simulink model "LTO"  (R2016b)
settings: Solver=VariableStepAuto  StartTime=0.0  StopTime=t24(end)  FixedStep=0.1  RelTol=1e-3
values from neighbouring files (symbols this model uses):
  Cpmap = [CpMapDis; CpMap]    [ltoMap.m]
  I0 = 0.0    (= 0)    [Main.m]
  Ich = 5    [Main.m]
  Idis = -15    [Main.m]
  Kch = 1.0    (= 1)    [Main.m]
  Kci = 1/(D2i^2*D3i)*(Tsig0*Lc)/(Tei^2)-Rtot    [Main.m]
  KI_cmp = KR_cmp/TI_cmp    [Main.m]
  KR_cmp = (1/Rb)*(Tsigc/D2c/Tec - 1)    [Main.m]
  Lc = 0.7e-3    (= 0.0007)    [Main.m]
  P0 = 1e-1*eye(2,2)    [Main.m]
  QChg = 33.0873    [Main.m]
  Qk = [qk11 0; 0 qk22]    [Main.m]
  Qmax24Chg = 32.9569    [Main.m]
  Rc = 0.05    [Main.m]
  rk = 1e1    (= 10)    [Main.m]
  Rpmap = [RpMapDis; RpMap]    [ltoMap.m]
  T = 0.01    [Main.m]
  Tacq = 1    [Main.m]
  Tch = 1e-3    (= 0.001)    [Main.m]
  Tci = (D3i*D2i^2*Tei^3*Kci)/(Tsig0*Lc)    [Main.m]
  Tfilt = 4e-3    (= 0.004)    [Main.m]
  uc0 = 0.0    (= 0)    [Main.m]
  Udc0 = 4    [Main.m]
undefined symbols (not defined in the file or in its folder): DiscIntNeverNeededParam, dUocdT_map, T_map, xi_map
libraries: dspmtrx3 x1, simulink x1, fuzblock x1
settings Model: Creator=user  LastModifiedBy=user

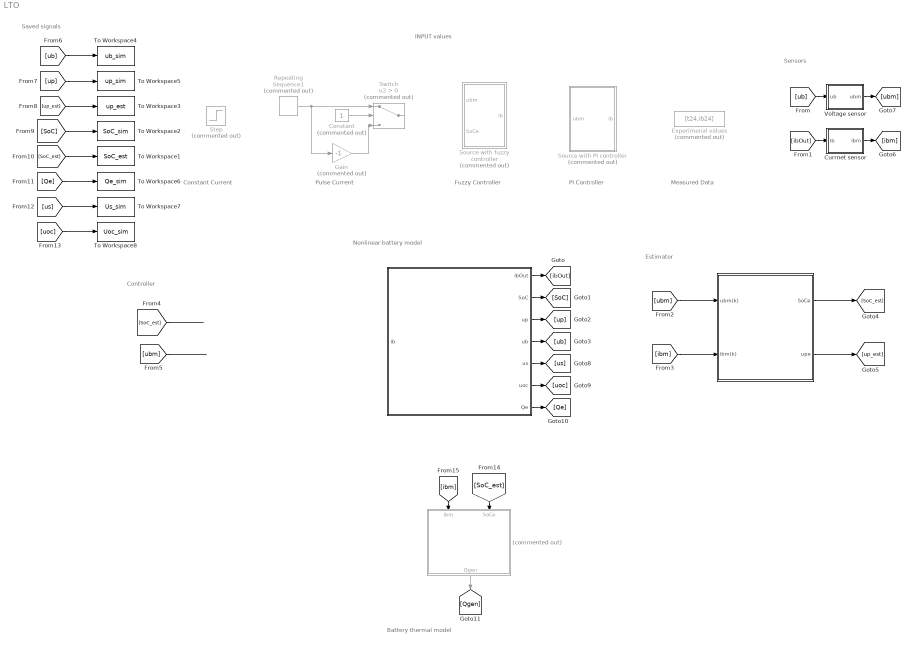
== system LTO ==
  note: Nonlinear battery model
  note: Constant Current
  note: Pulse Current
  note: Fuzzy Controller
  note: PI Controller
  note: Sensors
  note: Saved signals
  note: Measured Data
  note: INPUT values
  note: Estimator
  note: Battery thermal model
  note: Controller
  " " : Subsystem
  "  " : Subsystem  Commented=on
  "   " : Subsystem
  Constant : Constant  Commented=on
  Currnet sensor : Subsystem
  Experimenal values : FromWorkspace  Commented=on  VariableName=[t24,ib24]  SampleTime=Tacq
  Gain : Gain  Commented=on  Gain=-1
  Repeating Sequence1 : simulink/Sources/Repeating Sequence  Commented=on  rep_seq_t=[0 225 (225+2^(-40)) 300]  rep_seq_y=[Idis Idis Ich Ich]
  "Source with fuzzy controller " : Subsystem  Commented=on
  "Source with PI controller " : Subsystem  Commented=on
  Step : Step  Commented=on  After=30  SampleTime=0
  Switch : Switch  Commented=on  Criteria=u2 > Threshold
  To Workspace1 : ToWorkspace  VariableName=SoC_est  SampleTime=Tacq
  To Workspace2 : ToWorkspace  VariableName=SoC_sim  SampleTime=Tacq
  To Workspace3 : ToWorkspace  VariableName=up_est  SampleTime=Tacq
  To Workspace4 : ToWorkspace  VariableName=ub_sim  SampleTime=Tacq
  To Workspace5 : ToWorkspace  VariableName=up_sim  SampleTime=Tacq
  To Workspace6 : ToWorkspace  VariableName=Qe_sim  SampleTime=Tacq
  To Workspace7 : ToWorkspace  VariableName=Us_sim  SampleTime=Tacq
  To Workspace8 : ToWorkspace  VariableName=Uoc_sim  SampleTime=Tacq
  Voltage sensor : Subsystem
  wires:
  Constant/1 -> Switch/2
  Repeating Sequence1/1 -> Gain/1, Switch/1
  Gain/1 -> Switch/3
  " "/2(SoC) -> [SoC]
  " "/3(up) -> [up]
  " "/1("ibOut ") -> [ibOut]
  " "/4(ub) -> [ub]
  "   "/1(SoCe) -> [SoC_est]
  "   "/2(upe) -> [up_est]
  [ub] -> Voltage sensor/1(ub)
  [ibOut] -> Currnet sensor/1(ib)
  Voltage sensor/1("ubm ") -> [ubm]
  Currnet sensor/1("ibm ") -> [ibm]
  [ubm] -> "   "/1(ubm(k))
  [ibm] -> "   "/2(ibm(k))
  [ub] -> To Workspace4/1
  [up] -> To Workspace5/1
  [SoC_est] -> To Workspace1/1
  [up_est] -> To Workspace3/1
  [SoC] -> To Workspace2/1
  " "/5(us) -> [us]
  " "/6(uoc) -> [uoc]
  " "/7(Qe) -> [Qe]
  [Qe] -> To Workspace6/1
  [us] -> To Workspace7/1
  [uoc] -> To Workspace8/1
  [SoC_est] -> "  "/2(SoCe)
  [ibm] -> "  "/1(ibm)
  "  "/1(Qgen) -> [Qgen]
  [ubm] -> ?
  [SoC_est] -> ?

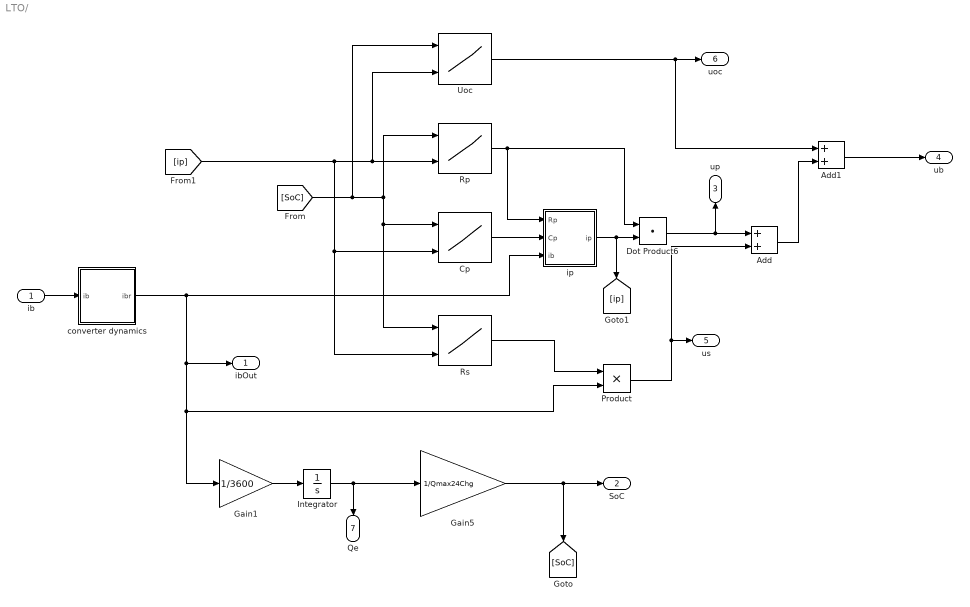
== system LTO/  ==
  ib : Inport
  Add : Sum
  Add1 : Sum
  Cp : Lookup2D  DialogController=Simulink.DDGSource  RowIndex=DxiMap  ColumnIndex=Imap  Table=Cpmap'  LookUpMeth=Interpolation-Use End Values
  Dot Product6 : DotProduct  InputSameDT=on  OutDataTypeStr=Inherit: Inherit via internal rule
  Gain1 : Gain  Gain=1/3600  OutDataTypeStr=Inherit: Same as input  ParamDataTypeStr=Inherit: Same as input
  Gain5 : Gain  Gain=1/Qmax24Chg  OutDataTypeStr=Inherit: Same as input  ParamDataTypeStr=Inherit: Same as input
  Integrator : Integrator
  Product : Product  RndMeth=Zero  OutDataTypeStr=Inherit: Same as first input
  Rp : Lookup2D  DialogController=Simulink.DDGSource  RowIndex=DxiMap  ColumnIndex=Imap  Table=Rpmap'  LookUpMeth=Interpolation-Use End Values  SaturateOnIntegerOverflow=on
  Rs : Lookup2D  DialogController=Simulink.DDGSource  RowIndex=DxiMap  ColumnIndex=Imap  Table=Rsmap'  LookUpMeth=Interpolation-Use End Values
      settings: LockScale=on
  Uoc : Lookup2D  DialogController=Simulink.DDGSource  RowIndex=DxiMap  ColumnIndex=Imap  Table=Uocmap'  SaturateOnIntegerOverflow=on
  converter dynamics : Subsystem
  ip : Subsystem
  "ibOut " : Outport
  SoC : Outport  Port=2
  up : Outport  Port=3
  ub : Outport  Port=4
  us : Outport  Port=5
  uoc : Outport  Port=6
  Qe : Outport  Port=7
  wires:
  Rs/1 -> Product/1
  Gain1/1 -> Integrator/1
  Gain5/1 -> [SoC], SoC/1
  ib/1 -> converter dynamics/1(ib)
  Integrator/1 -> Qe/1, Gain5/1
  Add1/1 -> ub/1
  [ip] -> Rs/2, Cp/2, Uoc/2, Rp/2
  [SoC] -> Uoc/1, Rs/1, Cp/1, Rp/1
  ip/1(ip) -> [ip], Dot Product6/2
  Cp/1 -> ip/2(Cp)
  Product/1 -> us/1, Add/2
  Uoc/1 -> Add1/1, uoc/1
  Add/1 -> Add1/2
  Dot Product6/1 -> Add/1, up/1
  Rp/1 -> ip/1(Rp), Dot Product6/1
  converter dynamics/1(ibr) -> ip/3(ib), "ibOut "/1, Product/2, Gain1/1

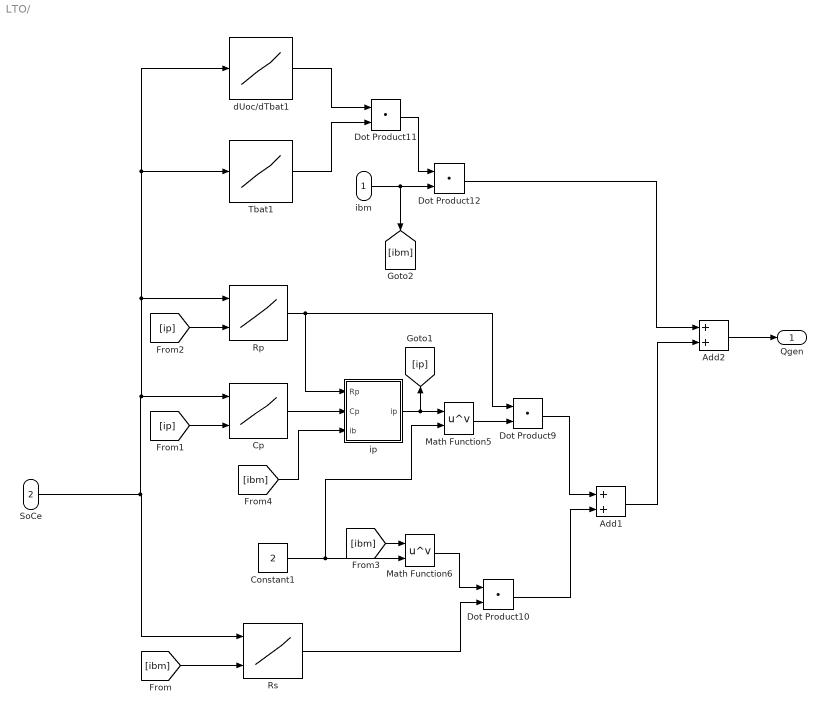
== system LTO/   ==
  ibm : Inport
  SoCe : Inport  Port=2
  Add1 : Sum
  Add2 : Sum
  Constant1 : Constant  Value=2
  Cp : Lookup2D  DialogController=Simulink.DDGSource  RowIndex=DxiMap  ColumnIndex=Imap  Table=Cpmap'  LookUpMeth=Interpolation-Use End Values
  Dot Product{9..12} (4 alike) : DotProduct  InputSameDT=on  OutDataTypeStr=Inherit: Inherit via internal rule
  Math Function5 : Math  Operator=pow  SaturateOnIntegerOverflow=on
  Math Function6 : Math  Operator=pow  SaturateOnIntegerOverflow=on
  Rp : Lookup2D  DialogController=Simulink.DDGSource  RowIndex=DxiMap  ColumnIndex=Imap  Table=Rpmap'  LookUpMeth=Interpolation-Use End Values  SaturateOnIntegerOverflow=on
  Rs : Lookup2D  DialogController=Simulink.DDGSource  RowIndex=DxiMap  ColumnIndex=Imap  Table=Rsmap'  LookUpMeth=Interpolation-Use End Values
      settings: LockScale=on
  Tbat1 : Lookup_n-D  NumberOfTableDimensions=1  BreakpointsForDimension1=xi_map  Table=T_map  InternalRulePriority=Speed  RndMeth=Simplest  InputSameDT=on
  dUoc/dTbat1 : Lookup_n-D  NumberOfTableDimensions=1  BreakpointsForDimension1=xi_map  Table=dUocdT_map  InternalRulePriority=Speed  RndMeth=Simplest  InputSameDT=on
  ip : Subsystem
  Qgen : Outport
  wires:
  [ip] -> Cp/2
  SoCe/1 -> Tbat1/1, dUoc/dTbat1/1, Rp/1, Cp/1, Rs/1
  Cp/1 -> ip/2(Cp)
  Rp/1 -> ip/1(Rp), Dot Product9/1
  ip/1(ip) -> [ip], Math Function5/1
  Math Function5/1 -> Dot Product9/2
  Constant1/1 -> Math Function5/2, Math Function6/2
  Math Function6/1 -> Dot Product10/1
  Rs/1 -> Dot Product10/2
  Dot Product9/1 -> Add1/1
  Dot Product10/1 -> Add1/2
  ibm/1 -> Dot Product12/2, [ibm]
  dUoc/dTbat1/1 -> Dot Product11/1
  Tbat1/1 -> Dot Product11/2
  Dot Product11/1 -> Dot Product12/1
  Dot Product12/1 -> Add2/1
  Add1/1 -> Add2/2
  Add2/1 -> Qgen/1
  [ibm] -> Rs/2
  [ip] -> Rp/2
  [ibm] -> Math Function6/1
  [ibm] -> ip/3(ib)

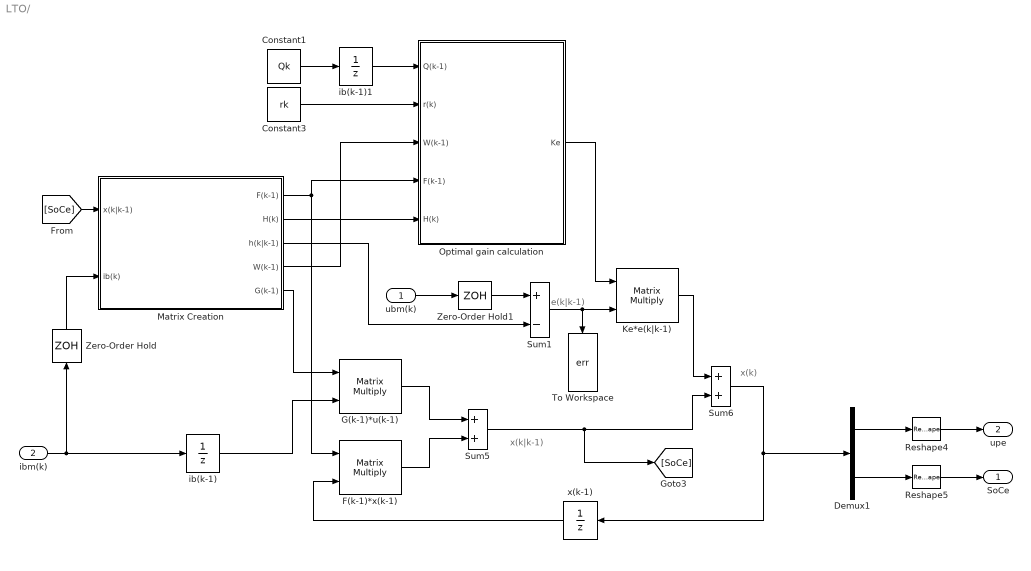
== system LTO/    ==
  note: x(k)
  note: e(k|k-1)
  note: x(k|k-1)
  ubm(k) : Inport
  ibm(k) : Inport  Port=2
  Constant1 : Constant  Value=Qk
  Constant3 : Constant  Value=rk
  Demux1 : Demux  Outputs=2
  F(k-1)*x(k-1) : Product  Multiplication=Matrix(*)  SampleTime=T  RndMeth=Zero
  G(k-1)*u(k-1) : Product  Multiplication=Matrix(*)  SampleTime=T  RndMeth=Zero
  Ke*e(k|k-1) : Product  Multiplication=Matrix(*)  SampleTime=T  RndMeth=Zero
  Matrix Creation : Subsystem
  Optimal gain calculation : Subsystem
  Reshape4 : Reshape
  Reshape5 : Reshape
  Sum1 : Sum  Inputs=+-  SampleTime=T  SaturateOnIntegerOverflow=on  InputSameDT=on  OutDataTypeStr=Inherit: Same as first input
  Sum5 : Sum  SampleTime=T  SaturateOnIntegerOverflow=on  InputSameDT=on  OutDataTypeStr=Inherit: Same as first input
  Sum6 : Sum  SampleTime=T  SaturateOnIntegerOverflow=on  InputSameDT=on  OutDataTypeStr=Inherit: Same as first input
  To Workspace : ToWorkspace  VariableName=err  SampleTime=-1
  Zero-Order Hold : ZeroOrderHold  SampleTime=T
  Zero-Order Hold1 : ZeroOrderHold  SampleTime=T
  ib(k-1) : UnitDelay  SampleTime=T
  ib(k-1)1 : UnitDelay  SampleTime=T
  x(k-1) : UnitDelay  InitialCondition=[0.265;0.15]  SampleTime=T
  SoCe : Outport
  upe : Outport  Port=2
  wires:
  ubm(k)/1 -> Zero-Order Hold1/1
  ibm(k)/1 -> ib(k-1)/1, Zero-Order Hold/1
  ib(k-1)/1 -> G(k-1)*u(k-1)/2
  G(k-1)*u(k-1)/1 -> Sum5/1
  F(k-1)*x(k-1)/1 -> Sum5/2
  Sum5/1 -> [SoCe], Sum6/2
  Sum6/1 -> x(k-1)/1, Demux1/1
  x(k-1)/1 -> F(k-1)*x(k-1)/2
  Zero-Order Hold1/1 -> Sum1/1
  Matrix Creation/3(h(k|k-1)) -> Sum1/2
  Sum1/1 -> To Workspace/1, Ke*e(k|k-1)/2
  Ke*e(k|k-1)/1 -> Sum6/1
  Reshape5/1 -> SoCe/1
  Reshape4/1 -> upe/1
  Matrix Creation/2(H(k)) -> Optimal gain calculation/5(H(k))
  Constant3/1 -> Optimal gain calculation/2(r(k))
  Constant1/1 -> ib(k-1)1/1
  Optimal gain calculation/1(Ke) -> Ke*e(k|k-1)/1
  Demux1/1 -> Reshape4/1
  Demux1/2 -> Reshape5/1
  Matrix Creation/5(G(k-1)) -> G(k-1)*u(k-1)/1
  Matrix Creation/1(F(k-1)) -> F(k-1)*x(k-1)/1, Optimal gain calculation/4(F(k-1))
  Matrix Creation/4(W(k-1)) -> Optimal gain calculation/3(W(k-1))
  Zero-Order Hold/1 -> Matrix Creation/2(ib(k))
  [SoCe] -> Matrix Creation/1(x(k|k-1))
  ib(k-1)1/1 -> Optimal gain calculation/1(Q(k-1))

== system LTO/Currnet sensor ==
  ib : Inport
  Gain : Gain  Gain=1/Tfilt  SaturateOnIntegerOverflow=on  OutDataTypeStr=Inherit: Same as input  ParamDataTypeStr=Inherit: Same as input
  Integrator : Integrator
  Sum : Sum  Inputs=+-  SaturateOnIntegerOverflow=on  InputSameDT=on  OutDataTypeStr=Inherit: Same as first input
  "ibm " : Outport
  wires:
  Sum/1 -> Gain/1
  Gain/1 -> Integrator/1
  Integrator/1 -> "ibm "/1, Sum/2
  ib/1 -> Sum/1

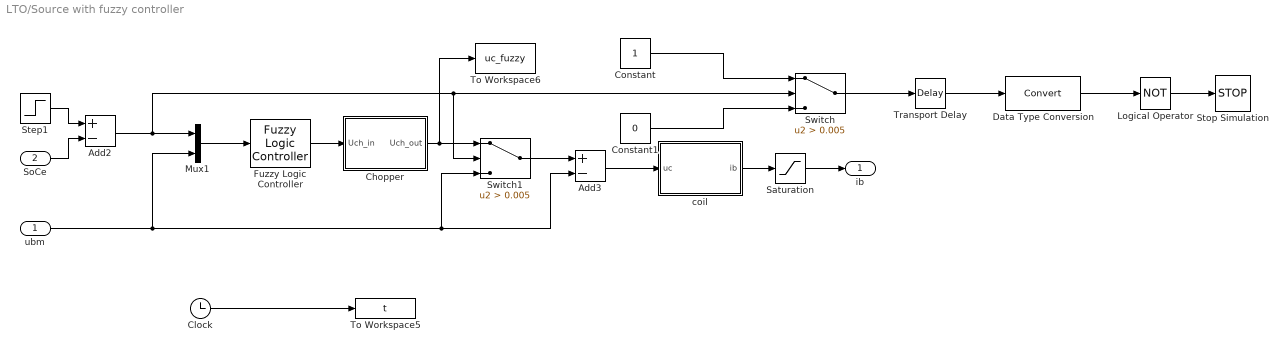
== system LTO/Source with fuzzy controller  ==
  ubm : Inport
  "SoCe " : Inport  Port=2
  Add2 : Sum  Inputs=+-
  Add3 : Sum  Inputs=+-
  Chopper : Subsystem
  Clock : Clock
  Constant : Constant
  Constant1 : Constant  Value=0
  Data Type Conversion : DataTypeConversion
  Fuzzy Logic Controller : fuzblock/Fuzzy Logic  Controller  fis='SoCcontroller'
  Logical Operator : Logic  Operator=NOT  AllPortsSameDT=off  OutDataTypeStr=boolean
  Mux1 : Mux  Inputs=2
  Saturation : Saturate  UpperLimit=30  LowerLimit=-30
  Step1 : Step  Time=0  SampleTime=0
  Stop Simulation : Stop
  Switch : Switch  Criteria=u2 > Threshold  Threshold=0.005
  Switch1 : Switch  Criteria=u2 > Threshold  Threshold=0.005
  To Workspace5 : ToWorkspace  VariableName=t  SampleTime=Tacq
  To Workspace6 : ToWorkspace  VariableName=uc_fuzzy  SampleTime=Tacq
  Transport Delay : TransportDelay  DelayTime=30  InitialOutput=1  BufferSize=64320
  coil : Subsystem
  "ib " : Outport
  wires:
  "SoCe "/1 -> Add2/2
  Add3/1 -> coil/1(uc)
  Add2/1 -> Switch1/2, Switch/2, Mux1/1
  Fuzzy Logic Controller/1 -> Chopper/1(Uch_in)
  Mux1/1 -> Fuzzy Logic Controller/1
  Step1/1 -> Add2/1
  coil/1(ib) -> Saturation/1
  ubm/1 -> Mux1/2, Switch1/3, Add3/2
  Clock/1 -> To Workspace5/1
  Chopper/1(Uch_out) -> To Workspace6/1, Switch1/1
  Switch1/1 -> Add3/1
  Constant/1 -> Switch/1
  Constant1/1 -> Switch/3
  Data Type Conversion/1 -> Logical Operator/1
  Switch/1 -> Transport Delay/1
  Logical Operator/1 -> Stop Simulation/1
  Transport Delay/1 -> Data Type Conversion/1
  Saturation/1 -> "ib "/1

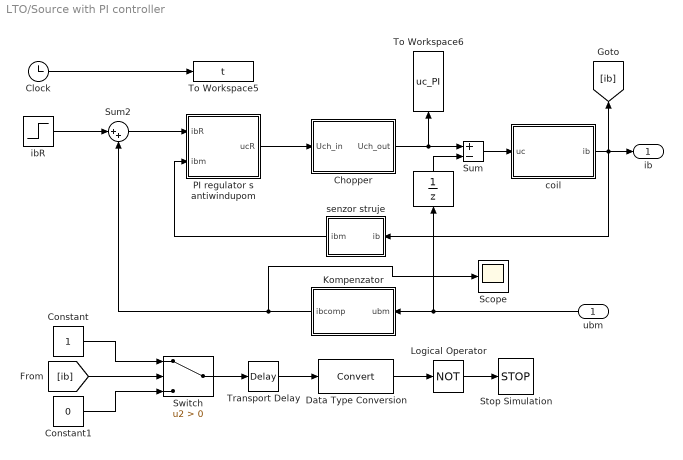
== system LTO/Source with PI controller  ==
  ubm : Inport
  " " : UnitDelay  SampleTime=T
  Chopper : Subsystem
  Clock : Clock
  Constant : Constant
  Constant1 : Constant  Value=0
  Data Type Conversion : DataTypeConversion
  "Kompenzator " : Subsystem
  Logical Operator : Logic  Operator=NOT  AllPortsSameDT=off  OutDataTypeStr=boolean
  PI regulator s antiwindupom : Subsystem
  Scope : Scope
  Stop Simulation : Stop
  Sum : Sum  Inputs=+-  SaturateOnIntegerOverflow=on  InputSameDT=on  OutDataTypeStr=Inherit: Same as first input
  Sum2 : Sum  Inputs=|++
  Switch : Switch  Criteria=u2 > Threshold
  To Workspace5 : ToWorkspace  VariableName=t  SampleTime=Tacq
  To Workspace6 : ToWorkspace  VariableName=uc_PI  SampleTime=Tacq
  Transport Delay : TransportDelay  DelayTime=30  InitialOutput=1  BufferSize=64320
  coil : Subsystem
  ibR : Step  Time=0  After=20  SampleTime=0
  senzor struje : Subsystem
  ib : Outport
  wires:
  ibR/1 -> Sum2/1
  "Kompenzator "/1(ibcomp) -> Scope/1, Sum2/2
  Sum2/1 -> PI regulator s antiwindupom/1(ibR)
  PI regulator s antiwindupom/1(ucR) -> Chopper/1(Uch_in)
  ubm/1 -> "Kompenzator "/1(ubm), " "/1
  senzor struje/1(ibm) -> PI regulator s antiwindupom/2(ibm)
  Clock/1 -> To Workspace5/1
  Chopper/1(Uch_out) -> Sum/1, To Workspace6/1
  coil/1(ib) -> senzor struje/1(ib), ib/1, [ib]
  Constant/1 -> Switch/1
  Constant1/1 -> Switch/3
  Data Type Conversion/1 -> Logical Operator/1
  Switch/1 -> Transport Delay/1
  Logical Operator/1 -> Stop Simulation/1
  Transport Delay/1 -> Data Type Conversion/1
  [ib] -> Switch/2
  Sum/1 -> coil/1(uc)
  " "/1 -> Sum/2

== system LTO/Voltage sensor ==
  ub : Inport
  Gain : Gain  Gain=1/Tfilt  SaturateOnIntegerOverflow=on  OutDataTypeStr=Inherit: Same as input  ParamDataTypeStr=Inherit: Same as input
  Integrator : Integrator
  Sum : Sum  Inputs=+-  SaturateOnIntegerOverflow=on  InputSameDT=on  OutDataTypeStr=Inherit: Same as first input
  "ubm " : Outport
  wires:
  Sum/1 -> Gain/1
  Gain/1 -> Integrator/1
  Integrator/1 -> "ubm "/1, Sum/2
  ub/1 -> Sum/1

== system LTO/ /converter dynamics ==
  ib : Inport
  converter dynamics : TransferFcn  Denominator=[5 1]
  ibr : Outport
  wires:
  converter dynamics/1 -> ibr/1
  ib/1 -> converter dynamics/1

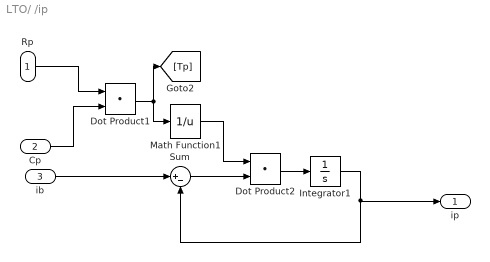
== system LTO/ /ip ==
  Rp : Inport
  Cp : Inport  Port=2
  ib : Inport  Port=3
  Dot Product1 : DotProduct  InputSameDT=on  OutDataTypeStr=Inherit: Inherit via internal rule
  Dot Product2 : DotProduct  InputSameDT=on  OutDataTypeStr=Inherit: Inherit via internal rule
  Integrator1 : Integrator
  Math Function1 : Math  Operator=reciprocal  SaturateOnIntegerOverflow=on
  Sum : Sum  Inputs=|+-
  ip : Outport
  wires:
  Integrator1/1 -> ip/1, Sum/2
  Sum/1 -> Dot Product2/2
  Cp/1 -> Dot Product1/2
  Math Function1/1 -> Dot Product2/1
  Dot Product2/1 -> Integrator1/1
  ib/1 -> Sum/1
  Rp/1 -> Dot Product1/1
  Dot Product1/1 -> Math Function1/1, [Tp]

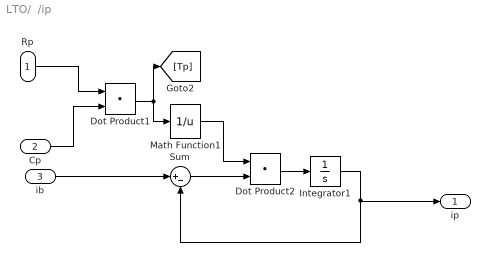
== system LTO/  /ip ==
  Rp : Inport
  Cp : Inport  Port=2
  ib : Inport  Port=3
  Dot Product1 : DotProduct  InputSameDT=on  OutDataTypeStr=Inherit: Inherit via internal rule
  Dot Product2 : DotProduct  InputSameDT=on  OutDataTypeStr=Inherit: Inherit via internal rule
  Integrator1 : Integrator
  Math Function1 : Math  Operator=reciprocal  SaturateOnIntegerOverflow=on
  Sum : Sum  Inputs=|+-
  ip : Outport
  wires:
  Integrator1/1 -> ip/1, Sum/2
  Sum/1 -> Dot Product2/2
  Cp/1 -> Dot Product1/2
  Math Function1/1 -> Dot Product2/1
  Dot Product2/1 -> Integrator1/1
  ib/1 -> Sum/1
  Rp/1 -> Dot Product1/1
  Dot Product1/1 -> Math Function1/1, [Tp]

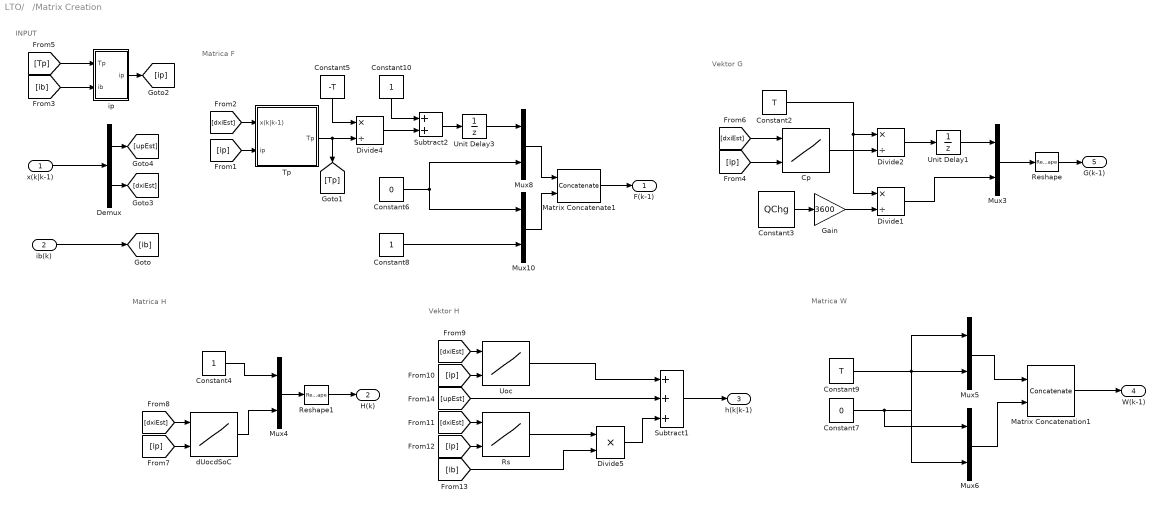
== system LTO/   /Matrix Creation ==
  note: Matrica F
  note: INPUT
  note: Vektor G
  note: Matrica H
  note: Vektor H
  note: Matrica W
  x(k|k-1) : Inport
  ib(k) : Inport  Port=2
  Constant10 : Constant
  Constant2 : Constant  Value=T
  Constant3 : Constant  Value=QChg
  Constant4 : Constant
  Constant5 : Constant  Value=-T
  Constant6 : Constant  Value=0
  Constant7 : Constant  Value=0
  Constant8 : Constant
  Constant9 : Constant  Value=T
  Cp : Lookup2D  DialogController=Simulink.DDGSource  RowIndex=DxiMap  ColumnIndex=Imap  Table=Cpmap'  LookUpMeth=Interpolation-Use End Values
  Demux : Demux  Outputs=2
  Divide1 : Product  Inputs=*/
  Divide2 : Product  Inputs=*/
  Divide4 : Product  Inputs=*/
  Divide5 : Product  Inputs=**
  Gain : Gain  Gain=3600
  Matrix Concatenate1 : Concatenate  Mode=Multidimensional array  ConcatenateDimension=2
  Matrix Concatenation1 : Concatenate  Mode=Multidimensional array  ConcatenateDimension=2
  Mux{3..6,8,10} (6 alike) : Mux  Inputs=2
  Reshape : Reshape  OutputDimensionality=Column vector (2-D)
  Reshape1 : Reshape  OutputDimensionality=Row vector (2-D)
  Rs : Lookup2D  DialogController=Simulink.DDGSource  RowIndex=DxiMap  ColumnIndex=Imap  Table=Rsmap'  LookUpMeth=Interpolation-Use End Values
      settings: LockScale=on
  Subtract1 : Sum  Inputs=+++
  Subtract2 : Sum
  Tp : Subsystem
  Unit Delay1 : UnitDelay  InitialCondition=T/mean(Cpmap(1,1001))  SampleTime=T
  Unit Delay3 : UnitDelay  InitialCondition=T/mean(Cpmap(1,1001).*Rpmap(1,1001))+1  SampleTime=T
  Uoc : Lookup2D  DialogController=Simulink.DDGSource  RowIndex=DxiMap  ColumnIndex=Imap  Table=Uocmap'  SaturateOnIntegerOverflow=on
  dUocdSoC : Lookup2D  DialogController=Simulink.DDGSource  RowIndex=DxiMap  ColumnIndex=Imap  Table=dUocdSoCmap'  LookUpMeth=Interpolation-Use End Values  SaturateOnIntegerOverflow=on
  ip : Subsystem
  F(k-1) : Outport
  H(k) : Outport  Port=2
  h(k|k-1) : Outport  Port=3
  W(k-1) : Outport  Port=4
  G(k-1) : Outport  Port=5
  wires:
  Cp/1 -> Divide2/2
  Divide2/1 -> Unit Delay1/1
  Constant2/1 -> Divide1/1, Divide2/1
  Mux3/1 -> Reshape/1
  Constant4/1 -> Mux4/1
  Mux4/1 -> Reshape1/1
  Reshape1/1 -> H(k)/1
  Mux5/1 -> Matrix Concatenation1/1
  Matrix Concatenation1/1 -> W(k-1)/1
  Mux6/1 -> Matrix Concatenation1/2
  Constant9/1 -> Mux6/2, Mux5/1
  Constant7/1 -> Mux6/1, Mux5/2
  Rs/1 -> Divide5/1
  Subtract1/1 -> h(k|k-1)/1
  Reshape/1 -> G(k-1)/1
  Unit Delay1/1 -> Mux3/1
  Constant3/1 -> Gain/1
  Gain/1 -> Divide1/2
  dUocdSoC/1 -> Mux4/2
  [ip] -> Cp/2
  [dxiEst] -> Cp/1
  ib(k)/1 -> [ib]
  Demux/1 -> [upEst]
  Demux/2 -> [dxiEst]
  [Tp] -> ip/1(Tp)
  ip/1(ip) -> [ip]
  [ib] -> ip/2(ib)
  x(k|k-1)/1 -> Demux/1
  Matrix Concatenate1/1 -> F(k-1)/1
  [dxiEst] -> Tp/1(x(k|k-1))
  [ip] -> Tp/2(ip)
  Constant8/1 -> Mux10/2
  Mux10/1 -> Matrix Concatenate1/2
  Tp/1(Tp) -> Divide4/2, [Tp]
  Unit Delay3/1 -> Mux8/1
  Subtract2/1 -> Unit Delay3/1
  Constant10/1 -> Subtract2/1
  Divide4/1 -> Subtract2/2
  Mux8/1 -> Matrix Concatenate1/1
  Constant6/1 -> Mux10/1, Mux8/2
  Constant5/1 -> Divide4/1
  Divide1/1 -> Mux3/2
  [ip] -> dUocdSoC/2
  [dxiEst] -> dUocdSoC/1
  [dxiEst] -> Uoc/1
  [ip] -> Uoc/2
  [dxiEst] -> Rs/1
  [ip] -> Rs/2
  [ib] -> Divide5/2
  Divide5/1 -> Subtract1/3
  Uoc/1 -> Subtract1/1
  [upEst] -> Subtract1/2

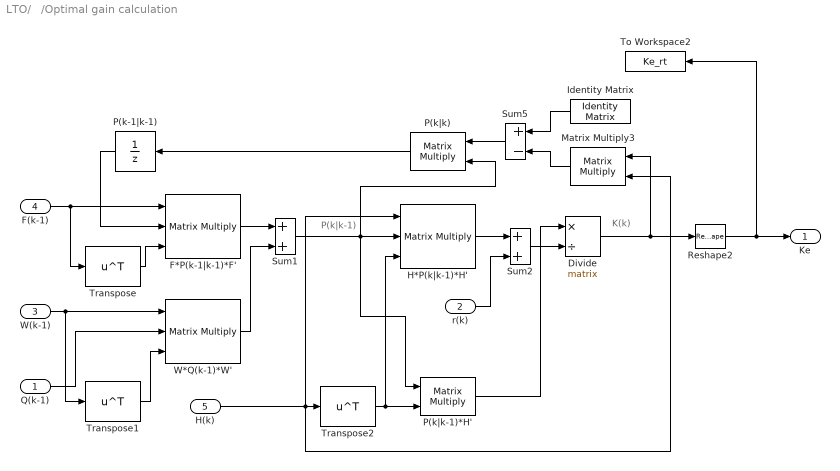
== system LTO/   /Optimal gain calculation ==
  note: P(k|k-1)
  note: K(k)
  Q(k-1) : Inport
  r(k) : Inport  Port=2
  W(k-1) : Inport  Port=3
  F(k-1) : Inport  Port=4
  H(k) : Inport  Port=5
  Divide : Product  Inputs=*/  Multiplication=Matrix(*)
  F*P(k-1|k-1)*F' : Product  Inputs=3  Multiplication=Matrix(*)
  H*P(k|k-1)*H' : Product  Inputs=3  Multiplication=Matrix(*)
  Identity Matrix : dspmtrx3/Identity Matrix  Inherit=off  N=2  Ts=T  dataType=double  isSigned=on  wordLen=16  udDataType=sfix(16)  fracBitsMode=Best precision  numFracBits=15  OutDataTypeStr=double  LastOutDataTypeStr=double
  Matrix Multiply3 : Product  Multiplication=Matrix(*)
  P(k-1|k-1) : UnitDelay  InitialCondition=P0  SampleTime=T
  P(k|k) : Product  Multiplication=Matrix(*)
  P(k|k-1)*H' : Product  Multiplication=Matrix(*)
  Reshape2 : Reshape
  Sum1 : Sum  SaturateOnIntegerOverflow=on  InputSameDT=on  OutDataTypeStr=Inherit: Same as first input
  Sum2 : Sum  SaturateOnIntegerOverflow=on  InputSameDT=on  OutDataTypeStr=Inherit: Same as first input
  Sum5 : Sum  Inputs=+-  SaturateOnIntegerOverflow=on  InputSameDT=on  OutDataTypeStr=Inherit: Same as first input
  To Workspace2 : ToWorkspace  VariableName=Ke_rt  SampleTime=Tacq
  Transpose : Math  Operator=transpose  SaturateOnIntegerOverflow=on
  Transpose1 : Math  Operator=transpose  SaturateOnIntegerOverflow=on
  Transpose2 : Math  Operator=transpose  SaturateOnIntegerOverflow=on
  W*Q(k-1)*W' : Product  Inputs=3  Multiplication=Matrix(*)
  Ke : Outport
  wires:
  Divide/1 -> Matrix Multiply3/1, Reshape2/1
  F(k-1)/1 -> Transpose/1, F*P(k-1|k-1)*F'/1
  W(k-1)/1 -> Transpose1/1, W*Q(k-1)*W'/1
  r(k)/1 -> Sum2/2
  Identity Matrix/1 -> Sum5/1
  Matrix Multiply3/1 -> Sum5/2
  P(k|k)/1 -> P(k-1|k-1)/1
  P(k-1|k-1)/1 -> F*P(k-1|k-1)*F'/2
  Transpose/1 -> F*P(k-1|k-1)*F'/3
  Transpose1/1 -> W*Q(k-1)*W'/3
  F*P(k-1|k-1)*F'/1 -> Sum1/1
  W*Q(k-1)*W'/1 -> Sum1/2
  Sum1/1 -> H*P(k|k-1)*H'/2, P(k|k-1)*H'/1, P(k|k)/2
  Transpose2/1 -> H*P(k|k-1)*H'/3, P(k|k-1)*H'/2
  H*P(k|k-1)*H'/1 -> Sum2/1
  Sum2/1 -> Divide/2
  P(k|k-1)*H'/1 -> Divide/1
  Sum5/1 -> P(k|k)/1
  Q(k-1)/1 -> W*Q(k-1)*W'/2
  Reshape2/1 -> To Workspace2/1, Ke/1
  H(k)/1 -> Transpose2/1, H*P(k|k-1)*H'/1, Matrix Multiply3/2

== system LTO/Source with fuzzy controller /Chopper ==
  Uch_in : Inport
  Gain : Gain  Gain=1/Tch  SaturateOnIntegerOverflow=on  OutDataTypeStr=Inherit: Same as input  ParamDataTypeStr=Inherit: Same as input
  Gain1 : Gain  Gain=Kch  SaturateOnIntegerOverflow=on  OutDataTypeStr=Inherit: Same as input  ParamDataTypeStr=Inherit: Same as input
  Integrator : Integrator
  Sum : Sum  Inputs=+-  SaturateOnIntegerOverflow=on  InputSameDT=on  OutDataTypeStr=Inherit: Same as first input
  Uch_out : Outport
  wires:
  Sum/1 -> Gain/1
  Gain1/1 -> Sum/1
  Uch_in/1 -> Gain1/1
  Gain/1 -> Integrator/1
  Integrator/1 -> Uch_out/1, Sum/2

== system LTO/Source with fuzzy controller /coil ==
  uc : Inport
  Gain : Gain  Gain=1/Lc  SaturateOnIntegerOverflow=on  OutDataTypeStr=Inherit: Same as input  ParamDataTypeStr=Inherit: Same as input
  Gain1 : Gain  Gain=Rc  SaturateOnIntegerOverflow=on  OutDataTypeStr=Inherit: Same as input  ParamDataTypeStr=Inherit: Same as input
  Integrator : Integrator
  Sum : Sum  Inputs=+-  SaturateOnIntegerOverflow=on  InputSameDT=on  OutDataTypeStr=Inherit: Same as first input
  ib : Outport
  wires:
  Integrator/1 -> ib/1, Gain1/1
  Gain/1 -> Integrator/1
  Sum/1 -> Gain/1
  uc/1 -> Sum/1
  Gain1/1 -> Sum/2

== system LTO/Source with PI controller /Chopper ==
  Uch_in : Inport
  Gain : Gain  Gain=1/Tch  SaturateOnIntegerOverflow=on  OutDataTypeStr=Inherit: Same as input  ParamDataTypeStr=Inherit: Same as input
  Gain1 : Gain  Gain=Kch  SaturateOnIntegerOverflow=on  OutDataTypeStr=Inherit: Same as input  ParamDataTypeStr=Inherit: Same as input
  Integrator : Integrator  InitialCondition=uc0
  Sum : Sum  Inputs=+-  SaturateOnIntegerOverflow=on  InputSameDT=on  OutDataTypeStr=Inherit: Same as first input
  Uch_out : Outport
  wires:
  Sum/1 -> Gain/1
  Gain1/1 -> Sum/1
  Uch_in/1 -> Gain1/1
  Gain/1 -> Integrator/1
  Integrator/1 -> Uch_out/1, Sum/2

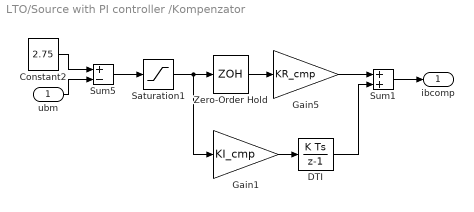
== system LTO/Source with PI controller /Kompenzator  ==
  ubm : Inport
  Constant2 : Constant  Value=2.75
  DTI : DiscreteIntegrator  SampleTime=T  ICPrevOutput=DiscIntNeverNeededParam  ICPrevScaledInput=DiscIntNeverNeededParam
  Gain1 : Gain  Gain=KI_cmp  SaturateOnIntegerOverflow=on  OutDataTypeStr=Inherit: Same as input  ParamDataTypeStr=Inherit: Same as input
  Gain5 : Gain  Gain=KR_cmp  SaturateOnIntegerOverflow=on  OutDataTypeStr=Inherit: Same as input  ParamDataTypeStr=Inherit: Same as input
  Saturation1 : Saturate  UpperLimit=0  LowerLimit=-0.3
  Sum1 : Sum  SaturateOnIntegerOverflow=on  InputSameDT=on  OutDataTypeStr=Inherit: Same as first input
  Sum5 : Sum  Inputs=+-  SaturateOnIntegerOverflow=on  InputSameDT=on  OutDataTypeStr=Inherit: Same as first input
  Zero-Order Hold : ZeroOrderHold  SampleTime=T
  ibcomp : Outport
  wires:
  Zero-Order Hold/1 -> Gain5/1
  Sum5/1 -> Saturation1/1
  Saturation1/1 -> Zero-Order Hold/1, Gain1/1
  Constant2/1 -> Sum5/1
  ubm/1 -> Sum5/2
  Gain1/1 -> DTI/1
  DTI/1 -> Sum1/2
  Gain5/1 -> Sum1/1
  Sum1/1 -> ibcomp/1

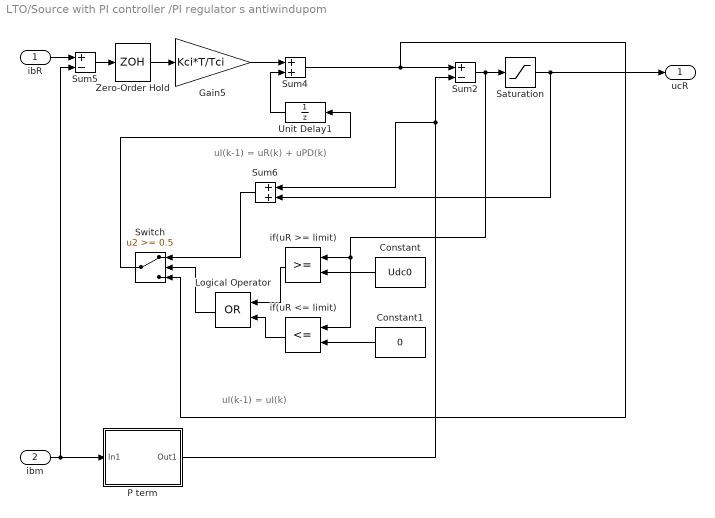
== system LTO/Source with PI controller /PI regulator s antiwindupom ==
  note: uI(k-1) = uI(k)
  note: uI(k-1) = uR(k) + uPD(k)
  ibR : Inport
  ibm : Inport  Port=2
  Constant : Constant  Value=Udc0
  Constant1 : Constant  Value=0
  Gain5 : Gain  Gain=Kci*T/Tci  SaturateOnIntegerOverflow=on  OutDataTypeStr=Inherit: Same as input  ParamDataTypeStr=Inherit: Same as input
  Logical Operator : Logic  Operator=OR
  "P term " : Subsystem
  Saturation : Saturate  UpperLimit=Udc0  LowerLimit=0
  Sum2 : Sum  Inputs=+-  SaturateOnIntegerOverflow=on  InputSameDT=on  OutDataTypeStr=Inherit: Same as first input
  Sum4 : Sum  SaturateOnIntegerOverflow=on  InputSameDT=on  OutDataTypeStr=Inherit: Same as first input
  Sum5 : Sum  Inputs=+-  SaturateOnIntegerOverflow=on  InputSameDT=on  OutDataTypeStr=Inherit: Same as first input
  Sum6 : Sum  SaturateOnIntegerOverflow=on  InputSameDT=on  OutDataTypeStr=Inherit: Same as first input
  Switch : Switch  Threshold=0.5  SaturateOnIntegerOverflow=on  InputSameDT=on
  Unit Delay1 : UnitDelay  InitialCondition=uc0 + Kci*I0  SampleTime=T
  Zero-Order Hold : ZeroOrderHold  SampleTime=T
  if(uR <= limit) : RelationalOperator  Operator=<=  RndMeth=Nearest  InputSameDT=on
  "if(uR >= limit) " : RelationalOperator  RndMeth=Nearest  InputSameDT=on
  ucR : Outport
  wires:
  Logical Operator/1 -> Switch/2
  if(uR <= limit)/1 -> Logical Operator/2
  "if(uR >= limit) "/1 -> Logical Operator/1
  Constant1/1 -> if(uR <= limit)/2
  ibm/1 -> Sum5/2, "P term "/1(In1)
  Zero-Order Hold/1 -> Gain5/1
  Sum5/1 -> Zero-Order Hold/1
  Switch/1 -> Unit Delay1/1
  Sum6/1 -> Switch/1
  Constant/1 -> "if(uR >= limit) "/2
  Sum4/1 -> Switch/3, Sum2/1
  Saturation/1 -> ucR/1, Sum6/2
  Sum2/1 -> if(uR <= limit)/1, "if(uR >= limit) "/1, Saturation/1
  ibR/1 -> Sum5/1
  Unit Delay1/1 -> Sum4/2
  Gain5/1 -> Sum4/1
  "P term "/1(Out1) -> Sum6/1, Sum2/2

== system LTO/Source with PI controller /coil ==
  uc : Inport
  Gain : Gain  Gain=1/Lc  SaturateOnIntegerOverflow=on  OutDataTypeStr=Inherit: Same as input  ParamDataTypeStr=Inherit: Same as input
  Gain1 : Gain  Gain=Rc  SaturateOnIntegerOverflow=on  OutDataTypeStr=Inherit: Same as input  ParamDataTypeStr=Inherit: Same as input
  Integrator : Integrator
  Sum : Sum  Inputs=+-  SaturateOnIntegerOverflow=on  InputSameDT=on  OutDataTypeStr=Inherit: Same as first input
  ib : Outport
  wires:
  Integrator/1 -> ib/1, Gain1/1
  Gain/1 -> Integrator/1
  Sum/1 -> Gain/1
  uc/1 -> Sum/1
  Gain1/1 -> Sum/2

== system LTO/Source with PI controller /senzor struje ==
  ib : Inport
  Gain : Gain  Gain=1/Tfilt  SaturateOnIntegerOverflow=on  OutDataTypeStr=Inherit: Same as input  ParamDataTypeStr=Inherit: Same as input
  Integrator : Integrator
  Sum : Sum  Inputs=+-  SaturateOnIntegerOverflow=on  InputSameDT=on  OutDataTypeStr=Inherit: Same as first input
  ibm : Outport
  wires:
  Sum/1 -> Gain/1
  Gain/1 -> Integrator/1
  Integrator/1 -> ibm/1, Sum/2
  ib/1 -> Sum/1

== system LTO/   /Matrix Creation/Tp ==
  x(k|k-1) : Inport
  ip : Inport  Port=2
  Cp1 : Lookup2D  DialogController=Simulink.DDGSource  RowIndex=DxiMap  ColumnIndex=Imap  Table=Cpmap'  LookUpMeth=Interpolation-Use End Values
  Product1 : Product  RndMeth=Zero  OutDataTypeStr=Inherit: Same as first input
  Rp : Lookup2D  DialogController=Simulink.DDGSource  RowIndex=DxiMap  ColumnIndex=Imap  Table=Rpmap'  LookUpMeth=Interpolation-Use End Values  SaturateOnIntegerOverflow=on
  Tp : Outport
  wires:
  ip/1 -> Cp1/2, Rp/2
  Cp1/1 -> Product1/2
  x(k|k-1)/1 -> Cp1/1, Rp/1
  Rp/1 -> Product1/1
  Product1/1 -> Tp/1

== system LTO/   /Matrix Creation/ip ==
  Tp : Inport
  ib : Inport  Port=2
  Dot Product2 : DotProduct  InputSameDT=on  OutDataTypeStr=Inherit: Inherit via internal rule
  Integrator1 : Integrator
  Math Function1 : Math  Operator=reciprocal  SaturateOnIntegerOverflow=on
  Sum : Sum  Inputs=|+-
  ip : Outport
  wires:
  Integrator1/1 -> ip/1, Sum/2
  Sum/1 -> Dot Product2/2
  Math Function1/1 -> Dot Product2/1
  Dot Product2/1 -> Integrator1/1
  ib/1 -> Sum/1
  Tp/1 -> Math Function1/1

== system LTO/Source with PI controller /PI regulator s antiwindupom/P term  ==
  In1 : Inport
  Gain1 : Gain  Gain=Kci  SaturateOnIntegerOverflow=on  OutDataTypeStr=Inherit: Same as input  ParamDataTypeStr=Inherit: Same as input
  Zero-Order Hold1 : ZeroOrderHold  SampleTime=T
  Out1 : Outport
  wires:
  In1/1 -> Zero-Order Hold1/1
  Zero-Order Hold1/1 -> Gain1/1
  Gain1/1 -> Out1/1
